simulink model "ASRUKF"  (R2024a)
settings: Solver=FixedStepAuto  StartTime=0.0  StopTime=16200  FixedStep=1  RelTol=1e-3
settings Model: Creator=yasha  LastModifiedBy=yasha

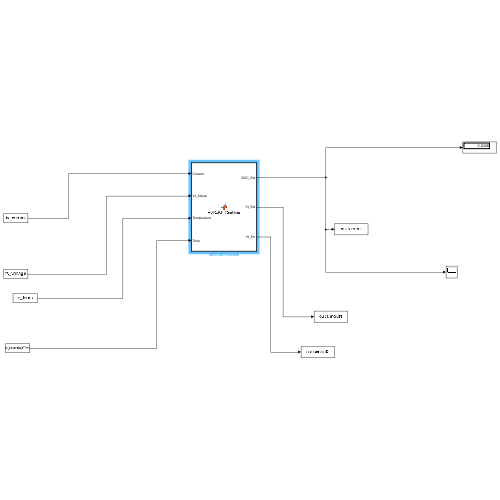
[thumbnail: Simulink's stored preview of the top-level diagram]
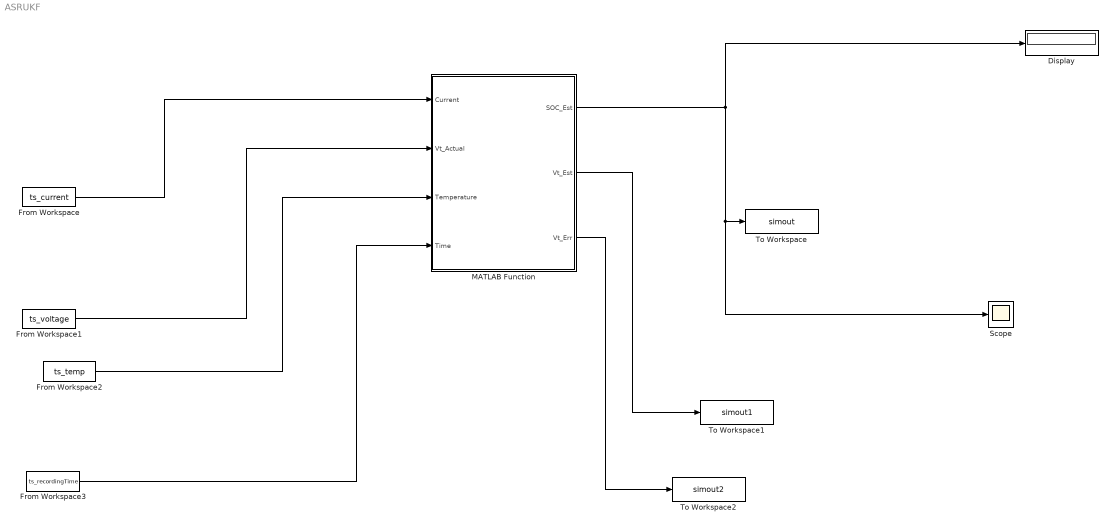
== system ASRUKF ==
  Display : Display
  From Workspace : FromWorkspace  VariableName=ts_current  SampleTime=1  Interpolate=off  OutputAfterFinalValue=Holding final value
  From Workspace1 : FromWorkspace  VariableName=ts_voltage  SampleTime=1  Interpolate=off  OutputAfterFinalValue=Holding final value
  From Workspace2 : FromWorkspace  VariableName=ts_temp  SampleTime=1  Interpolate=off  OutputAfterFinalValue=Holding final value
  From Workspace3 : FromWorkspace  VariableName=ts_recordingTime  SampleTime=1  Interpolate=off  OutputAfterFinalValue=Holding final value
  MATLAB Function : MATLAB Function  TreatAsAtomicUnit=on
  Scope : Scope
  To Workspace : ToWorkspace  VariableName=simout  SaveFormat=Timeseries  SampleTime=-1
  To Workspace1 : ToWorkspace  VariableName=simout1  SaveFormat=Timeseries  SampleTime=-1
  To Workspace2 : ToWorkspace  VariableName=simout2  SaveFormat=Timeseries  SampleTime=-1
  wires:
  From Workspace/1 -> MATLAB Function/1(Current)
  From Workspace1/1 -> MATLAB Function/2(Vt_Actual)
  From Workspace2/1 -> MATLAB Function/3(Temperature)
  From Workspace3/1 -> MATLAB Function/4(Time)
  MATLAB Function/1(SOC_Est) -> Scope/1, To Workspace/1, Display/1
  MATLAB Function/3(Vt_Err) -> To Workspace2/1
  MATLAB Function/2(Vt_Est) -> To Workspace1/1

== matlab function ASRUKF/MATLAB Function ==
  data: Current input; SOC_Est output; Vt_Actual input; Temperature input; Time input; Vt_Est output; Vt_Err output
function [SOC_Est, Vt_Est, Vt_Err] = ASRUKF_Realtime(Current, Vt_Actual, Temperature, Time)
%#codegen

% Persistent variables to maintain state between function calls
persistent x_hat S SQ SR ev_history innovation_count k_count
persistent SOC_Init QN eta deltaT SOCOCV dSOCOCV
persistent param_T param_SOC param_R0 param_R1 param_R2 param_C1 param_C2
persistent alpha beta kappa lambda w_m w_c b M SQ_min SR_min initialized

% Initialize on first call
if isempty(initialized)
    
    % Battery Parameters
    SOC_Init = 0.3;
    QN = 4.81 * 3600;
    eta = 1.0;
    deltaT = 1;
    
    % ASRUKF Parameters
    n = 3;
    alpha = 0.01;
    beta = 2;
    kappa = 3 - n;
    lambda = alpha^2 * (n + kappa) - n;
    
    % Weights
    w_m = zeros(2*n+1, 1);
    w_c = zeros(2*n+1, 1);
    w_m(1) = lambda/(n+lambda);
    w_c(1) = w_m(1) + (1 - alpha^2 + beta);
    for i = 2:2*n+1
        w_m(i) = 1/(2*(n+lambda));
        w_c(i) = w_m(i);
    end
    
    % Initial state and covariance
    x_hat = [SOC_Init; 0; 0];
    P_init = [0.25 0 0; 0 0.05 0; 0 0 0.05];
    S = chol(P_init, 'lower');
    
    % Process and measurement noise
    Q_init = [5e-4 0 0; 0 1.0e-6 0; 0 0 1.0e-6];
    SQ = chol(Q_init, 'lower');
    SR = sqrt(1.0e-4);
    
    % Adaptive parameters
    b = 0.95;
    M = 10;
    ev_history = zeros(M, 1);
    innovation_count = 0;
    k_count = 0;
    
    % Minimum noise bounds
    SQ_min = diag([1.0e-6, 1.0e-8, 1.0e-8]);
    SR_min = 1.0e-5;
    
    % *** YOUR ACTUAL BATTERY PARAMETERS ***
    % Temperature points
    param_T = [-10.0, -10.0, -10.0, -10.0, -10.0, -10.0, -10.0, -10.0, -10.0, -10.0, ...
               0.0, 0.0, 0.0, 0.0, 0.0, 0.0, 0.0, 0.0, 0.0, 0.0, ...
               10.0, 10.0, 10.0, 10.0, 10.0, 10.0, 10.0, 10.0, 10.0, 10.0, ...
               25.0, 25.0, 25.0, 25.0, 25.0, 25.0, 25.0, 25.0, 25.0, 25.0, ...
               40.0, 40.0, 40.0, 40.0, 40.0, 40.0, 40.0, 40.0, 40.0, 40.0];
    
    % SOC points
    param_SOC = [0.11, 0.16, 0.24, 0.29, 0.49, 0.49, 0.70, 0.77, 0.89, 0.99, ...
                 0.08, 0.12, 0.28, 0.30, 0.45, 0.57, 0.68, 0.79, 0.89, 1.00, ...
                 0.07, 0.15, 0.23, 0.33, 0.45, 0.56, 0.68, 0.78, 0.89, 0.99, ...
                 0.07, 0.14, 0.23, 0.34, 0.44, 0.55, 0.66, 0.77, 0.89, 1.00, ...
                 0.01, 0.08, 0.21, 0.26, 0.41, 0.52, 0.64, 0.76, 0.89, 0.99];
    
    % R0 parameter values
    param_R0 = [0.051018; 0.0332552; 0.0288058; 0.0250401; 0.0242543; 0.0218737; 0.021629; 0.0199578; 0.020999; 0.0208976; ...
                0.00100014; 0.0128431; 0.0157735; 0.0105689; 0.0128425; 0.0101624; 0.0107265; 0.0101553; 0.0105078; 0.0104174; ...
                0.0138462; 0.00895056; 0.00878031; 0.00783427; 0.00737131; 0.00684761; 0.00655256; 0.00659363; 0.00689802; 0.00668035; ...
                0.017425; 0.00936607; 0.00850813; 0.00783404; 0.00723289; 0.00671684; 0.00639564; 0.00633668; 0.00660493; 0.00641603; ...
                0.00472931; 0.00170684; 0.00242514; 0.0017591; 0.00194551; 0.00172803; 0.00165793; 0.0017522; 0.00177816; 0.00173403];
    
    % R1 parameter values
    param_R1 = [0.000490331; 0.000503898; 0.00050397; 0.000505462; 0.000505161; 0.00050718; 0.00050004; 0.000504438; 0.000499932; 0.000504727; ...
                0.00049907; 0.000497947; 0.000495452; 0.000506356; 0.000504828; 0.000504599; 0.000499319; 0.000505662; 0.000498598; 0.000497742; ...
                0.000517305; 0.000504511; 0.000504415; 0.000511754; 0.000496082; 0.000496362; 0.000501225; 0.000493715; 0.00050351; 0.000503348; ...
                0.000486022; 0.00050176; 0.000499248; 0.000496115; 0.000499789; 0.000495121; 0.000501191; 0.000501637; 0.000497013; 0.00050321; ...
                0.00053604; 0.000504197; 0.000514078; 0.000528667; 0.000490667; 0.000541283; 0.000528384; 0.000512774; 0.00051786; 0.000515144];
    
    % R2 parameter values
    param_R2 = [0.0005; 0.0005; 0.0005; 0.0005; 0.0005; 0.0005; 0.0005; 0.0005; 0.0005; 0.0005; ...
                0.000495631; 0.000484431; 0.000503443; 0.000496275; 0.00049695; 0.000498807; 0.000501132; 0.00049939; 0.000500443; 0.000501072; ...
                0.000499931; 0.0004919; 0.000522796; 0.000497236; 0.000498209; 0.000496461; 0.000497273; 0.000499376; 0.000503661; 0.000501774; ...
                0.000488772; 0.000497864; 0.000499846; 0.000495479; 0.000500232; 0.000502407; 0.000503902; 0.000504341; 0.000500666; 0.000492471; ...
                0.000535684; 0.00049106; 0.000507067; 0.000517108; 0.000511585; 0.000510458; 0.0005091; 0.000500386; 0.000530881; 0.000515451];
    
    % C1 parameter values
    param_C1 = [20384.5; 19885.4; 19667.2; 19681.5; 20230.5; 19693.8; 20364.9; 20252.1; 20201.2; 19848.7; ...
                20127.2; 20529.3; 20164.8; 19554.7; 19779; 19592; 20057.9; 19775; 19945.2; 20218.9; ...
                19295.1; 19973.9; 19997.2; 19539.1; 19976.5; 20060.4; 20076.2; 20439; 19953.1; 19871.6; ...
                20108.9; 19824.2; 19993.2; 20178.1; 20137.9; 20477.3; 20088.8; 19885.8; 20392.8; 20002; ...
                16732.2; 19566.2; 20344.4; 19175.1; 20262.9; 18447.3; 19359.5; 19619.2; 19398; 19575.6];
    
    % C2 parameter values
    param_C2 = [200000; 200000; 200000; 200000; 200000; 200000; 200000; 200000; 200000; 200000; ...
                201696; 207017; 199004; 202674; 200848; 202566; 198330; 200313; 199863; 201614; ...
                197944; 206282; 194454; 199967; 201208; 201695; 205114; 199978; 196708; 200137; ...
                203503; 204201; 200038; 202403; 200030; 198381; 198503; 198134; 199336; 199951; ...
                171880; 206800; 198967; 193860; 203645; 195065; 196021; 192824; 189489; 199164];
    
    % *** YOUR ACTUAL SOC-OCV DATA ***
    % SOC-OCV polynomial coefficients (order 6)
    SOCOCV = [-4.746665e+01, 1.649823e+02, -2.283789e+02, 1.610269e+02, -6.045348e+01, 1.166351e+01, 2.823836e+00];
    dSOCOCV = polyder(SOCOCV);
    
    initialized = true;
end

% Increment sample counter
k_count = k_count + 1;

% Current state
SOC = x_hat(1);
V1 = x_hat(2);
V2 = x_hat(3);

% Get battery parameters using nearest neighbor interpolation
% (since your data points are scattered, not on a regular grid)
distances = sqrt((param_SOC - SOC).^2 + ((param_T - Temperature)/50).^2);
[~, idx] = min(distances);

R0 = param_R0(idx);
R1 = param_R1(idx);
R2 = param_R2(idx);
C1 = param_C1(idx);
C2 = param_C2(idx);

% Calculate discrete-time parameters
Tau_1 = C1 * R1;
Tau_2 = C2 * R2;
a1 = exp(-deltaT/Tau_1);
a2 = exp(-deltaT/Tau_2);
b1 = R1 * (1 - exp(-deltaT/Tau_1));
b2 = R2 * (1 - exp(-deltaT/Tau_2));

% OCV calculation
OCV = polyval(SOCOCV, SOC);

% Calculate outputs
Vt_Est = OCV - R0*Current - V1 - V2;
SOC_Est = SOC;
Vt_Err = Vt_Actual - Vt_Est;

% Skip update for first sample
if k_count == 1
    return;
end

% ASRUKF Update Steps
n = 3;

% System matrices
A = [1, 0, 0; 0, a1, 0; 0, 0, a2];
B = [-(eta * deltaT/QN); b1; b2];

% Generate sigma points
sqrt_term = sqrt(n + lambda) * S;
chi = [x_hat, x_hat + sqrt_term, x_hat - sqrt_term];

% Time update
chi_pred = zeros(3, 2*n+1);
for i = 1:2*n+1
    chi_pred(:, i) = A * chi(:, i) + B * Current;
    chi_pred(1, i) = max(0.01, min(0.99, chi_pred(1, i))); % SOC bounds
end

% Predicted state mean
x_pred = zeros(3, 1);
for i = 1:2*n+1
    x_pred = x_pred + w_m(i) * chi_pred(:, i);
end

% Predicted covariance square root
X_dev = chi_pred(:, 2:end) - x_pred;
for i = 1:2*n
    X_dev(:, i) = sqrt(abs(w_c(i+1))) * X_dev(:, i);
end

[~, S_pred] = qr([X_dev, SQ]', 0);
S_pred = S_pred';

% Cholupdate for first sigma point
if w_c(1) >= 0
    S_pred = cholupdate(S_pred, sqrt(w_c(1)) * (chi_pred(:, 1) - x_pred), '+');
else
    S_pred = cholupdate(S_pred, sqrt(abs(w_c(1))) * (chi_pred(:, 1) - x_pred), '-');
end

% Measurement update
sqrt_term = sqrt(n + lambda) * S_pred;
chi_pred = [x_pred, x_pred + sqrt_term, x_pred - sqrt_term];

% Measurement prediction
z_pred = zeros(1, 2*n+1);
for i = 1:2*n+1
    soc_i = max(0.01, min(0.99, chi_pred(1, i)));
    v1_i = chi_pred(2, i);
    v2_i = chi_pred(3, i);
    
    % Get parameters for current sigma point
    distances_i = sqrt((param_SOC - soc_i).^2 + ((param_T - Temperature)/50).^2);
    [~, idx_i] = min(distances_i);
    R0_i = param_R0(idx_i);
    
    OCV_i = polyval(SOCOCV, soc_i);
    z_pred(i) = OCV_i - R0_i*Current - v1_i - v2_i;
end

% Predicted measurement mean
z_mean = 0;
for i = 1:2*n+1
    z_mean = z_mean + w_m(i) * z_pred(i);
end

% Calculate Kalman gain
Z_dev = z_pred(2:end) - z_mean;
for i = 1:2*n
    Z_dev(i) = sqrt(abs(w_c(i+1))) * Z_dev(i);
end

[~, Szz] = qr([Z_dev, SR]', 0);
Szz = Szz(1,1);

if w_c(1) >= 0
    Szz = cholupdate(Szz, sqrt(abs(w_c(1))) * (z_pred(1) - z_mean), '+');
else
    Szz = cholupdate(Szz, sqrt(abs(w_c(1))) * (z_pred(1) - z_mean), '-');
end

% Cross-covariance
Pxz = zeros(3, 1);
for i = 1:2*n+1
    Pxz = Pxz + w_c(i) * (chi_pred(:, i) - x_pred) * (z_pred(i) - z_mean);
end

% Kalman gain
K = Pxz / (Szz * Szz');

% State update
innovation = Vt_Actual - z_mean;
x_hat = x_pred + K * innovation;
x_hat(1) = max(0.01, min(0.99, x_hat(1))); % SOC bounds

% Covariance update
%try
    S = cholupdate(S_pred, K * Szz, '-');
%catch
    % Fallback to Joseph form
    %H_jacobian = [polyval(dSOCOCV, x_hat(1)), -1, -1];
    %I_KH = eye(3) - K * H_jacobian;
    %P_new = I_KH * (S_pred * S_pred') * I_KH' + K * (SR^2) * K';
    %P_new = P_new + 1e-8 * eye(3);
    %S = chol(P_new, 'lower');
%end

% Adaptive noise estimation
innovation_count = innovation_count + 1;

if innovation_count <= M
    ev_history(innovation_count) = innovation^2;
else
    ev_history = [ev_history(2:end); innovation^2];
end

if innovation_count >= M
    F_k = mean(ev_history);
    d_k = (1 - b^k_count)/(1 - b^(k_count+1));
    
    Q_factor = sqrt(F_k);
    SQ_new = diag([Q_factor*1e-3, Q_factor*1e-5, Q_factor*1e-5]) + SQ_min;
    SQ = (1 - d_k) * SQ + d_k * SQ_new;
    
    SR_new = sqrt(F_k) + SR_min;
    SR = (1 - d_k) * SR + d_k * SR_new;
end

% Update outputs with current estimates
SOC_Est = x_hat(1);
Vt_Est = OCV - R0*Current - x_hat(2) - x_hat(3);
Vt_Err = Vt_Actual - Vt_Est;

end
